simulink model "Visualization"  (R2026a)
settings: Solver=VariableStepAuto
undefined symbols (not defined in the file): ts_uav, waypoints
libraries: uavutilslib x1
settings Model: DataDictionary=QuadData.sldd  Creator=The MathWorks, Inc.  LastModifiedBy=The MathWorks, Inc.

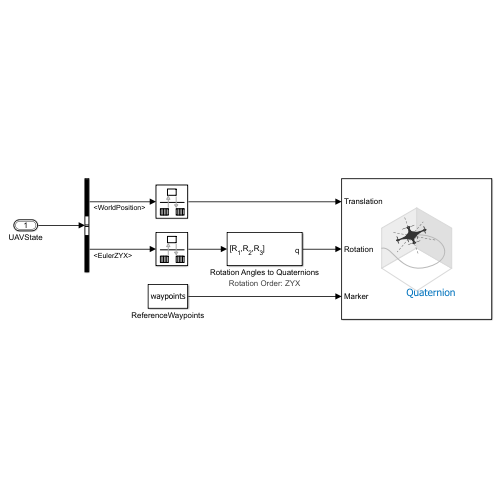
[thumbnail: Simulink's stored preview of the top-level diagram]
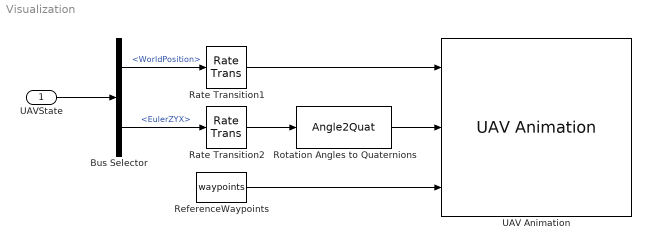
== system Visualization ==
  UAVState : Inport  OutDataTypeStr=Bus: MultirotorGuidanceStateBus  SampleTime=0
  Bus Selector : BusSelector  OutputSignals=WorldPosition,EulerZYX
  Rate Transition1 : RateTransition  OutPortSampleTime=0.1
  Rate Transition2 : RateTransition  OutPortSampleTime=0.1
  ReferenceWaypoints : Constant  Value=waypoints  SampleTime=ts_uav
  Rotation Angles to Quaternions : Angle2Quat
      settings: AttributesFormatString=Rotation Order: %<rotationOrder>
  UAV Animation : uavutilslib/UAV Animation  NumUAV=1  DynamicUAVConfig=off  UAVType=Multirotor  UAVSize=1  UAVColor=[1 0 0]  UAVTrajectoryAlpha=1  AlwaysShowAnimation=on  AxisLimits=[-Inf Inf;-Inf Inf;-Inf Inf]  TrajectoryBufferSize=100000  InertialZDirection=Down  RotationFormat=Quaternion  DrawMarkers=on  SampleTime=-1
  wires:
  Rate Transition1/1 -> UAV Animation/1
  Rate Transition2/1 -> Rotation Angles to Quaternions/1
  Rotation Angles to Quaternions/1 -> UAV Animation/2
  UAVState/1 -> Bus Selector/1
  Bus Selector/1 -> Rate Transition1/1  "<WorldPosition>"
  Bus Selector/2 -> Rate Transition2/1  "<EulerZYX>"
  ReferenceWaypoints/1 -> UAV Animation/3
